simulink model "onboard_control"  (Simulink 9.2)
settings: Solver=FixedStepAuto  StartTime=0.0  StopTime=10.0  RelTol=1e-3
undefined symbols (not defined in the file or in its folder): inner_ac, inner_angle_h, inner_arc, inner_rate_h, inner_thrust_lim, inner_thrust_min, inner_yc, inner_yrc
settings Model: Creator=sebbe  LastModifiedBy=sebbe
settings DataIOCC: LimitDataPoints=off  SaveFormat=Dataset  SignalLoggingSaveFormat=Dataset
settings OptimizationCC: LifeSpan=auto
settings DebuggingCC: UnderspecifiedInitializationDetection=Simplified  MergeDetectMultiDrivingBlocksExec=error  FcnCallInpInsideContextMsg=error  StateNameClashWarn=none  SFUnexpectedBacktrackingDiag=error  SFNoUnconditionalDefaultTransitionDiag=error  SFExecutionAtInitializationDiag=warning
settings HardwareCC: ProdBitPerPointer=64  ProdBitPerSizeT=64  ProdBitPerPtrDiffT=64  ProdLargestAtomicFloat=Float  ProdIntDivRoundTo=Zero  ProdEndianess=LittleEndian  ProdWordSize=64  ProdHWDeviceType=Intel->x86-64 (Windows64)
settings ModelReferenceCC: PropagateSignalLabelsOutOfModel=on
settings SFSimCC: SimUseLocalCustomCode=on
settings RTWCC: RTWUseLocalCustomCode=on
settings CodeAppCC: StateflowObjectComments=off
settings GRTTargetCC: TargetLangStandard=C99 (ISO)  GeneratePreprocessorConditionals=Use local settings  CombineOutputUpdateFcns=on  GRTInterface=off
settings ConfigComp: CovMetricSettings=dwe  CovHtmlReporting=off  CovSaveCumulativeToWorkspaceVar=off  CovSaveSingleToWorkspaceVar=off  CovExternalEMLEnable=on

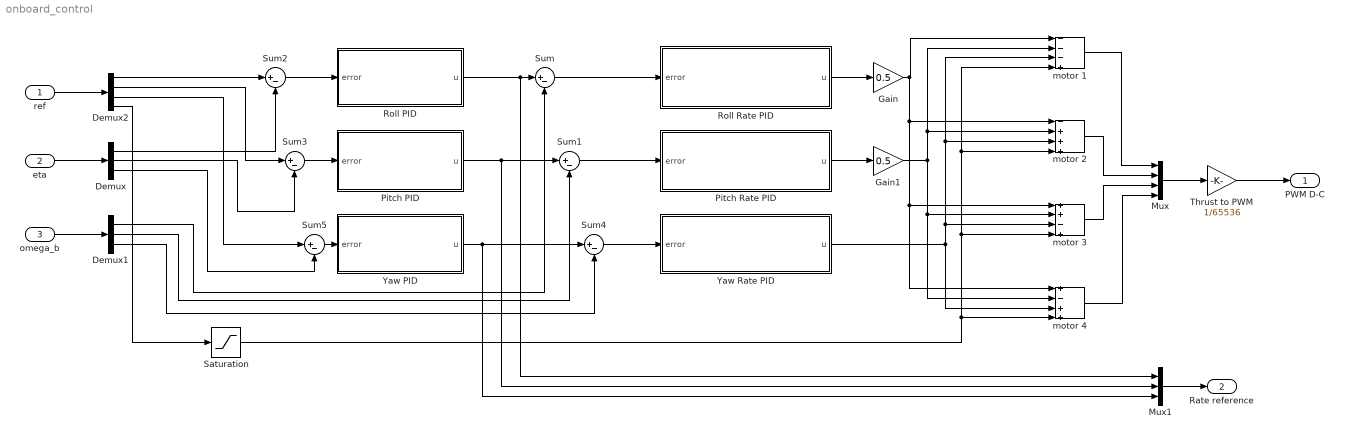
== system onboard_control ==
  ref : Inport
  eta : Inport  Port=2
  omega_b : Inport  Port=3  PortDimensions=[3]
  Demux : Demux  Outputs=3
  Demux1 : Demux  Outputs=3
  Demux2 : Demux
  Gain : Gain  Gain=0.5
  Gain1 : Gain  Gain=0.5
  Mux : Mux
  Mux1 : Mux  Inputs=3
  Pitch PID : MATLAB Function  TreatAsAtomicUnit=on  SystemSampleTime=inner_rate_h
  Pitch Rate PID : MATLAB Function  TreatAsAtomicUnit=on  SystemSampleTime=inner_rate_h
  Roll PID : MATLAB Function  TreatAsAtomicUnit=on  SystemSampleTime=inner_rate_h
  Roll Rate PID : MATLAB Function  TreatAsAtomicUnit=on  SystemSampleTime=inner_rate_h
  Saturation : Saturate  UpperLimit=65535*inner_thrust_lim  LowerLimit=65535*inner_thrust_min
  Sum{,1..5} (6 alike) : Sum  Inputs=|+-
  Thrust to PWM : Gain  Gain=1/65536
  Yaw PID : MATLAB Function  TreatAsAtomicUnit=on  SystemSampleTime=inner_rate_h
  Yaw Rate PID : MATLAB Function  TreatAsAtomicUnit=on  SystemSampleTime=inner_rate_h
  motor 1 : Sum  Inputs=-|-|-|+
  motor 2 : Sum  Inputs=-|+|+|+
  motor 3 : Sum  Inputs=+|+|-|+
  motor 4 : Sum  Inputs=+|-|+|+
  PWM D-C : Outport
  Rate reference : Outport  Port=2
  wires:
  eta/1 -> Demux/1
  Demux1/3 -> Sum4/2
  Demux1/2 -> Sum1/2
  Demux1/1 -> Sum/2
  Yaw PID/1(u) -> Sum4/1, Mux1/3
  Sum/1 -> Roll Rate PID/1(error)
  Sum1/1 -> Pitch Rate PID/1(error)
  Gain1/1 -> motor 4/2, motor 3/2, motor 2/2, motor 1/2
  Yaw Rate PID/1(u) -> motor 4/3, motor 3/3, motor 1/3, motor 2/3
  Demux2/4 -> Saturation/1
  Gain/1 -> motor 4/1, motor 3/1, motor 2/1, motor 1/1
  Mux/1 -> Thrust to PWM/1
  motor 1/1 -> Mux/1
  motor 2/1 -> Mux/2
  motor 3/1 -> Mux/3
  motor 4/1 -> Mux/4
  Demux/1 -> Sum2/2
  ref/1 -> Demux2/1
  Demux2/1 -> Sum2/1
  Demux2/2 -> Sum3/1
  Demux2/3 -> Sum5/1
  Demux/2 -> Sum3/2
  Demux/3 -> Sum5/2
  Sum5/1 -> Yaw PID/1(error)
  Thrust to PWM/1 -> PWM D-C/1
  Pitch Rate PID/1(u) -> Gain1/1
  Sum4/1 -> Yaw Rate PID/1(error)
  Mux1/1 -> Rate reference/1
  Roll Rate PID/1(u) -> Gain/1
  omega_b/1 -> Demux1/1
  Saturation/1 -> motor 4/4, motor 3/4, motor 2/4, motor 1/4
  Sum2/1 -> Roll PID/1(error)
  Roll PID/1(u) -> Mux1/1, Sum/1
  Sum3/1 -> Pitch PID/1(error)
  Pitch PID/1(u) -> Mux1/2, Sum1/1

== matlab function Pitch PID ==
  data: error input double; u output double; inner_ac parameter double; inner_angle_h parameter double
function u = pitch_PID(error, inner_ac, inner_angle_h)
    % Initialization of persistent variables
    persistent pers
    if isempty(pers)
        pers.prev_error = 0;
        pers.integ = 0;
        pers.delay_e = [0 0 0];
    end
    
    [u, pers] = inner_PID(error, inner_ac, inner_angle_h, pers);
end

== matlab function Roll Rate PID ==
  data: error input double; u output double; inner_arc parameter double; inner_rate_h parameter double
function u = roll_PID_rate(error, inner_arc, inner_rate_h)
    % Initialization of persistent variables
    persistent pers
    if isempty(pers)
        pers.prev_error = 0;
        pers.integ = 0;
        pers.delay_e = [0 0 0];
    end
    
    [u, pers] = inner_PID(error, inner_arc, inner_rate_h, pers);
end

== matlab function Pitch Rate PID ==
  data: error input double; u output double; inner_arc parameter double; inner_rate_h parameter double
function u = pitch_PID_rate(error, inner_arc, inner_rate_h)
    % Initialization of persistent variables
    persistent pers
    if isempty(pers)
        pers.prev_error = 0;
        pers.integ = 0;
        pers.delay_e = [0 0 0];
    end
    
    [u, pers] = inner_PID(error, inner_arc, inner_rate_h, pers);
end

== matlab function Yaw Rate PID ==
  data: error input double; u output double; inner_yrc parameter double; inner_rate_h parameter double
function u = yaw_PID_rate(error, inner_yrc, inner_rate_h)
    % Initialization of persistent variables
    persistent pers
    if isempty(pers)
        pers.prev_error = 0;
        pers.integ = 0;
        pers.delay_e = [0 0 0];
    end
    
    [u, pers] = inner_PID(error, inner_yrc, inner_rate_h, pers);
end

== matlab function Roll PID ==
  data: error input double; u output double; inner_ac parameter double; inner_angle_h parameter double
function u = roll_PID(error, inner_ac, inner_angle_h)
    % Initialization of persistent variables
    persistent pers
    if isempty(pers)
        pers.prev_error = 0;
        pers.integ = 0;
        pers.delay_e = [0 0 0];
    end
    
    [u, pers] = inner_PID(error, inner_ac, inner_angle_h, pers);
end

== matlab function Yaw PID ==
  data: error input double; u output double; inner_yc parameter double; inner_angle_h parameter double
function u = yaw_PID(error, inner_yc, inner_angle_h)
    % Initialization of persistent variables
    persistent pers
    if isempty(pers)
        pers.prev_error = 0;
        pers.integ = 0;
        pers.delay_e = [0 0 0];
    end
    
    [u, pers] = inner_PID(error, inner_yc, inner_angle_h, pers);
end
